simulink model "R19_Modelo_nolineal_1GDL_2021"  (R2019b)
settings: Solver=VariableStepAuto  StartTime=0.0  StopTime=5  FixedStep=T  RelTol=1e-3
values from neighbouring files (symbols this model uses):
  g = 9.81    [CONTROL_1GDL_BANCADA.m]
  k1 = 100386.825573    [COEFICIENTES_HEMS.mat]
  k2 = 80.9361649813    [COEFICIENTES_HEMS.mat]
  k3 = -5115.69918255    [COEFICIENTES_HEMS.mat]
  k4 = -499734.269698    [COEFICIENTES_HEMS.mat]
  m = 122/6    (= 20.3333333333)    [CONTROL_1GDL_BANCADA.m]
  p1 = 0.100560433707    [COEFICIENTES_HEMS.mat]
  p2 = 0.00460149528539    [COEFICIENTES_HEMS.mat]
  z0 = 17.5*1e-3    (= 0.0175)    [CONTROL_1GDL_BANCADA.m]
settings Model: Creator=EDMAOR  LastModifiedBy=CARRARO2
settings SFSimCC: CustomCodeUndefinedFunction=UseInterfaceOnly

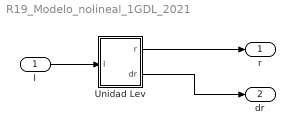
== system R19_Modelo_nolineal_1GDL_2021 ==
  I : Inport
  Unidad Lev : Subsystem
  r : Outport  VectorParamsAs1DForOutWhenUnconnected=off
  dr : Outport  Port=2  VectorParamsAs1DForOutWhenUnconnected=off
  wires:
  Unidad Lev/1(r) -> r/1
  Unidad Lev/2(dr) -> dr/1
  I/1 -> Unidad Lev/1(I)

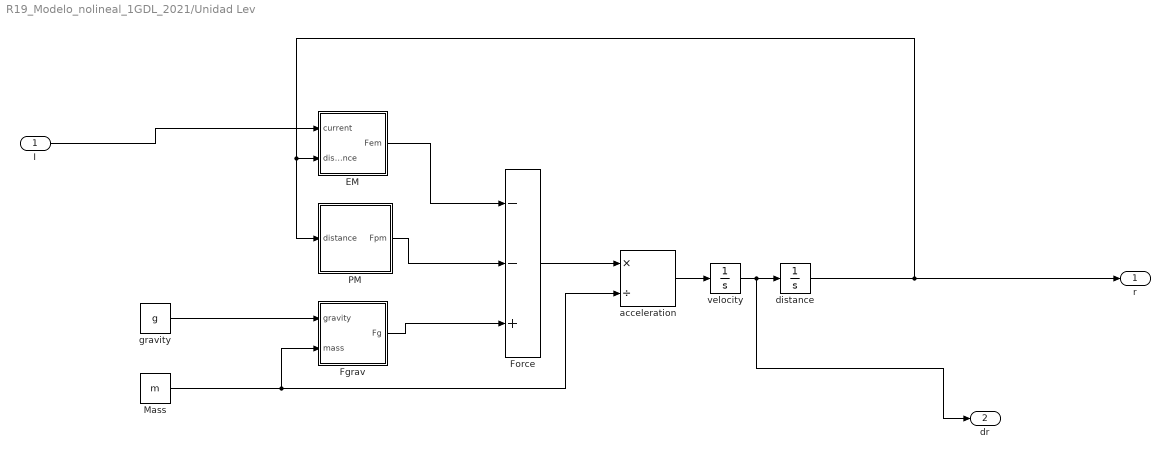
== system R19_Modelo_nolineal_1GDL_2021/Unidad Lev ==
  I : Inport
  EM : Subsystem
  Fgrav : Subsystem
  Force : Sum  Inputs=--+
  Mass : Constant  Value=m
  PM : Subsystem
  acceleration : Product  Inputs=*/
  distance : Integrator  InitialCondition=z0
  gravity : Constant  Value=g
  velocity : Integrator
  r : Outport  VectorParamsAs1DForOutWhenUnconnected=off
  dr : Outport  Port=2  VectorParamsAs1DForOutWhenUnconnected=off
  wires:
  Force/1 -> acceleration/1
  EM/1(Fem) -> Force/1
  Fgrav/1(Fg) -> Force/3
  gravity/1 -> Fgrav/1(gravity)
  acceleration/1 -> velocity/1
  Mass/1 -> Fgrav/2(mass), acceleration/2
  I/1 -> EM/1(current)
  PM/1(Fpm) -> Force/2
  velocity/1 -> dr/1, distance/1
  distance/1 -> PM/1(distance), EM/2(distance), r/1

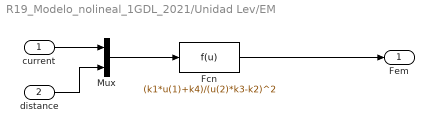
== system R19_Modelo_nolineal_1GDL_2021/Unidad Lev/EM ==
  current : Inport
  distance : Inport  Port=2
  Fcn : Fcn  Expr=(k1*u(1)+k4)/(u(2)*k3-k2)^2
  Mux : Mux  Inputs=2
  Fem : Outport  VectorParamsAs1DForOutWhenUnconnected=off
  wires:
  current/1 -> Mux/1
  distance/1 -> Mux/2
  Mux/1 -> Fcn/1
  Fcn/1 -> Fem/1

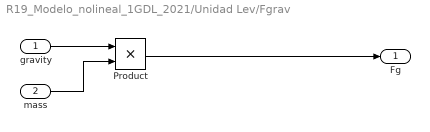
== system R19_Modelo_nolineal_1GDL_2021/Unidad Lev/Fgrav ==
  gravity : Inport
  mass : Inport  Port=2
  Product : Product
  Fg : Outport  VectorParamsAs1DForOutWhenUnconnected=off
  wires:
  Product/1 -> Fg/1
  gravity/1 -> Product/1
  mass/1 -> Product/2

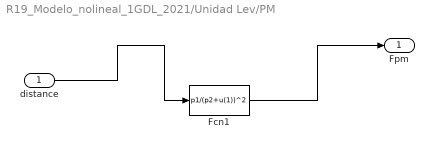
== system R19_Modelo_nolineal_1GDL_2021/Unidad Lev/PM ==
  distance : Inport
  Fcn1 : Fcn  Expr=p1/(p2+u(1))^2
  Fpm : Outport  VectorParamsAs1DForOutWhenUnconnected=off
  wires:
  distance/1 -> Fcn1/1
  Fcn1/1 -> Fpm/1
